simulink model "x231040036_a1"  (R2024a)
settings: Solver=ode3  StartTime=0.0  StopTime=0.2  RelTol=1e-3
InitFcn:
  | fs=1550
  | Ts=1/1550
libraries: spsIGBTDiodeLib x6, spsVoltageMeasurementLib x5, spsSeriesRLCBranchLib x3, simulink x1, spsDCVoltageSourceLib x1, spsGroundLib x1, spsRMSLib x1, spspowerguiLib x1
settings Model: Creator=aayus  LastModifiedBy=bpven
settings DataIOCC: SaveFormat=StructureWithTime  SaveTime=off  ReturnWorkspaceOutputs=off
settings RTWCC: GPUComputeCapability=3.5

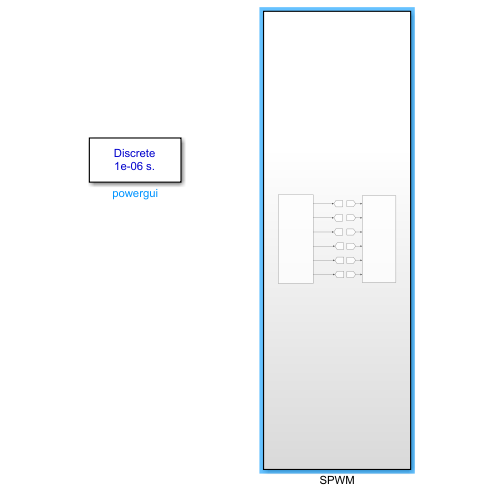
[thumbnail: Simulink's stored preview of the top-level diagram]
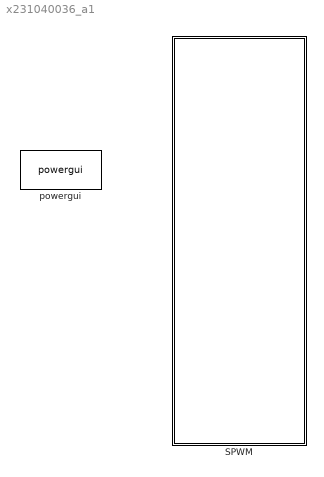
== system x231040036_a1 ==
  SPWM : Subsystem
  powergui : spspowerguiLib/powergui  Priority=1  SimulationMode=Discrete  SampleTime=1e-6  frequency=60  Iterations=50  frequencyindice=0  Pbase=100e6  ErrMax=1e-4  UnitsV=kV  UnitsW=MW  buscounter=0  FunctionMessages=off  echomessages=off  EnableUseOfTLC=off  CurrentSourceSwitches=off  DisableSnubberDevices=off  DisableRonSwitches=off  DisableVfSwitches=off  DisplayEquations=off  AutomaticDiscreteSolvers=off  SolverType=Tustin/Backward Euler (TBE)  Interpol=off  ExternalGateDelay=off  methode=off  Ts=100  x0status=blocks  SPID=on  SwTol=0  HookPort=off  NonlinearTolerance=1e-4  nMaxIteration=100  ContinueOnMaxIteration=off  RestoreLinks=warning  ResistiveCurrentMeasurement=off  Frange=[0:2:500]  Ylog=off  Xlog=on  ShowGrid=off  save=off  variable=ZData  structure=0  ZoomFFT=off  StartTime=0.0  cycles=1  DisplayStyle=1  fundamental=60  FreqAxis=off  MaxFrequency=1000  frequencyindicesteady=1  RmsSteady=1  display=off

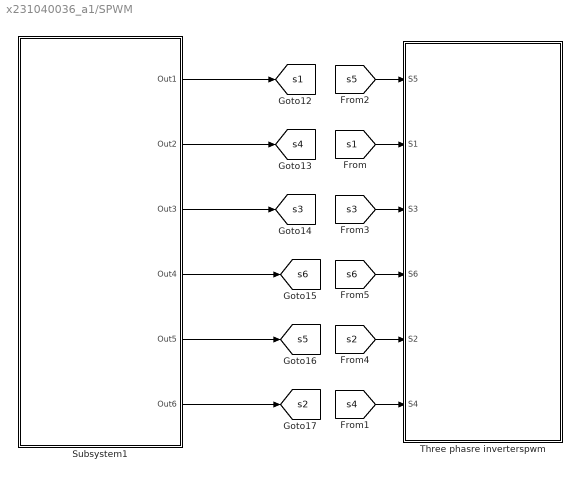
== system x231040036_a1/SPWM ==
  Subsystem1 : Subsystem
  Three phasre inverterspwm : Subsystem
  tag scope: s1=global, s2=global, s3=global, s4=global, s5=global, s6=global
  wires:
  [s2] -> Three phasre inverterspwm/5(S2)
  [s1] -> Three phasre inverterspwm/2(S1)
  [s5] -> Three phasre inverterspwm/1(S5)
  Subsystem1/4(Out4) -> [s6]
  Subsystem1/3(Out3) -> [s3]
  [s6] -> Three phasre inverterspwm/4(S6)
  [s4] -> Three phasre inverterspwm/6(S4)
  [s3] -> Three phasre inverterspwm/3(S3)
  Subsystem1/6(Out6) -> [s2]
  Subsystem1/2(Out2) -> [s4]
  Subsystem1/5(Out5) -> [s5]
  Subsystem1/1(Out1) -> [s1]

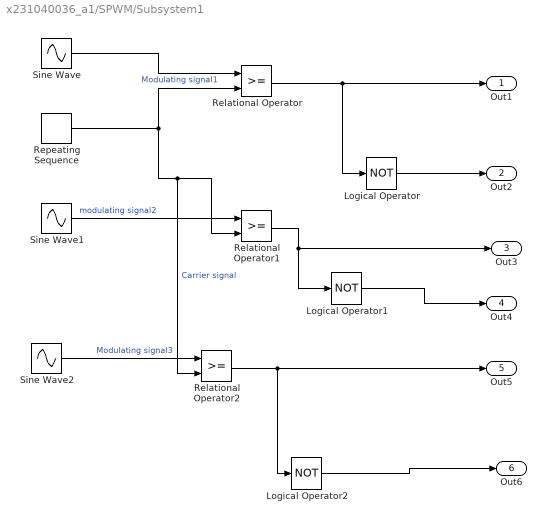
== system x231040036_a1/SPWM/Subsystem1 ==
  Logical Operator : Logic  Operator=NOT  AllPortsSameDT=off  OutDataTypeStr=boolean
  Logical Operator1 : Logic  Operator=NOT  AllPortsSameDT=off  OutDataTypeStr=boolean
  Logical Operator2 : Logic  Operator=NOT  AllPortsSameDT=off  OutDataTypeStr=boolean
  Relational Operator : RelationalOperator  OutDataTypeStr=boolean  RndMeth=Simplest  InputSameDT=off
  Relational Operator1 : RelationalOperator  OutDataTypeStr=boolean  RndMeth=Simplest  InputSameDT=off
  Relational Operator2 : RelationalOperator  OutDataTypeStr=boolean  RndMeth=Simplest  InputSameDT=off
  Repeating Sequence : simulink/Sources/Repeating Sequence  rep_seq_t=[0 0.5 1]*(1/1550)  rep_seq_y=[-1 1 -1]
  Sine Wave : Sin  Frequency=2*pi*50  SampleTime=0
  Sine Wave1 : Sin  Frequency=2*pi*50  Phase=2*pi/3  SampleTime=0
  Sine Wave2 : Sin  Frequency=2*pi*50  Phase=4*pi/3  SampleTime=0
  Out1 : Outport
  Out2 : Outport  Port=2
  Out3 : Outport  Port=3
  Out4 : Outport  Port=4
  Out5 : Outport  Port=5
  Out6 : Outport  Port=6
  wires:
  Repeating Sequence/1 -> Relational Operator/2, Relational Operator2/2, Relational Operator1/2  "Carrier signal"
  Logical Operator2/1 -> Out6/1
  Relational Operator/1 -> Out1/1, Logical Operator/1
  Relational Operator2/1 -> Out5/1, Logical Operator2/1
  Relational Operator1/1 -> Out3/1, Logical Operator1/1
  Sine Wave2/1 -> Relational Operator2/1  "Modulating signal3"
  Sine Wave1/1 -> Relational Operator1/1  "modulating signal2"
  Sine Wave/1 -> Relational Operator/1  "Modulating signal1"
  Logical Operator/1 -> Out2/1
  Logical Operator1/1 -> Out4/1

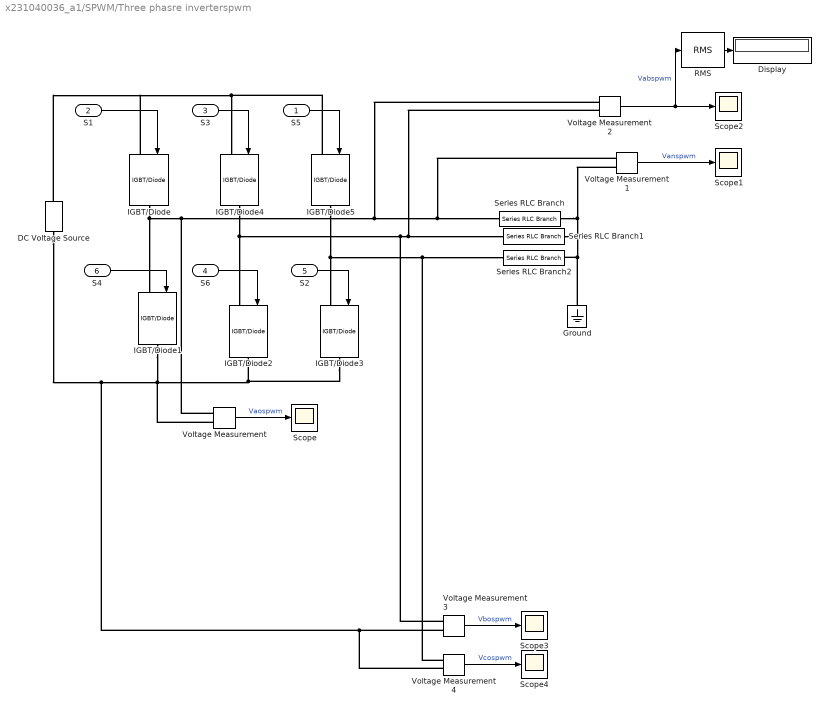
== system x231040036_a1/SPWM/Three phasre inverterspwm ==
  S5 : Inport
  S1 : Inport  Port=2
  S3 : Inport  Port=3
  S6 : Inport  Port=4
  S2 : Inport  Port=5
  S4 : Inport  Port=6
  DC Voltage Source : spsDCVoltageSourceLib/DC Voltage Source  Amplitude=400  Measurements=None
  Display : Display
  Ground : spsGroundLib/Ground  LConnTagsString=a
  IGBT/Diode{,1..5} (6 alike) : spsIGBTDiodeLib/IGBT//Diode  Ron=1e-3  Rs=1e5  Cs=inf  Measurements=off
  RMS : spsRMSLib/RMS  TrueRMS=on  Freq=50  RMSInit=120  Ts=0
  Scope{,1..4} (5 alike) : Scope
  Series RLC Branch : spsSeriesRLCBranchLib/Series RLC Branch  LConnTagsString=__new0  RConnTagsString=__new0  BranchType=R  Resistance=1  Inductance=1e-3  SetiL0=off  InitialCurrent=0  Capacitance=1e-6  Setx0=off  InitialVoltage=0  Measurements=None
  Series RLC Branch1 : spsSeriesRLCBranchLib/Series RLC Branch  LConnTagsString=__new0  RConnTagsString=__new0  BranchType=R  Resistance=1  Inductance=1e-3  SetiL0=off  InitialCurrent=0  Capacitance=1e-6  Setx0=off  InitialVoltage=0  Measurements=None
  Series RLC Branch2 : spsSeriesRLCBranchLib/Series RLC Branch  LConnTagsString=__new0  RConnTagsString=__new0  BranchType=R  Resistance=1  Inductance=1e-3  SetiL0=off  InitialCurrent=0  Capacitance=1e-6  Setx0=off  InitialVoltage=0  Measurements=None
  Voltage Measurement{,1..4} (5 alike) : spsVoltageMeasurementLib/Voltage Measurement  PhasorSimulation=off  OutputType=Complex  PSBequivalent=0
  wires:
  Voltage Measurement1/1 -> Scope1/1  "Vanspwm"
  Voltage Measurement/1 -> Scope/1  "Vaospwm"
  Voltage Measurement2/1 -> RMS/1, Scope2/1  "Vabspwm"
  S3/1 -> IGBT/Diode4/1
  S5/1 -> IGBT/Diode5/1
  S2/1 -> IGBT/Diode3/1
  S4/1 -> IGBT/Diode1/1
  S6/1 -> IGBT/Diode2/1
  S1/1 -> IGBT/Diode/1
  RMS/1 -> Display/1
  Voltage Measurement4/1 -> Scope4/1  "Vcospwm"
  Voltage Measurement3/1 -> Scope3/1  "Vbospwm"
  connections:
  Voltage Measurement3/LConn2 -- IGBT/Diode3/RConn1 -- IGBT/Diode2/RConn1 -- Voltage Measurement/LConn2 -- IGBT/Diode1/RConn1 -- DC Voltage Source/LConn1 -- Voltage Measurement4/LConn2
  IGBT/Diode5/RConn1 -- IGBT/Diode3/LConn1 -- Series RLC Branch2/LConn1 -- Voltage Measurement4/LConn1
  IGBT/Diode5/LConn1 -- DC Voltage Source/RConn1 -- IGBT/Diode/LConn1 -- IGBT/Diode4/LConn1
  IGBT/Diode4/RConn1 -- IGBT/Diode2/LConn1 -- Voltage Measurement3/LConn1 -- Voltage Measurement2/LConn2 -- Series RLC Branch1/LConn1
  IGBT/Diode/RConn1 -- Voltage Measurement/LConn1 -- Voltage Measurement2/LConn1 -- Voltage Measurement1/LConn1 -- Series RLC Branch/LConn1 -- IGBT/Diode1/LConn1
  Series RLC Branch/RConn1 -- Ground/LConn1 -- Series RLC Branch2/RConn1 -- Series RLC Branch1/RConn1 -- Voltage Measurement1/LConn2
